simulink model "missionplanning"  (R2020b)
settings: Solver=FixedStepAuto  StartTime=0.0  StopTime=10.0  FixedStep=0.1  RelTol=1e-3
values from neighbouring files (symbols this model uses):
  A_DB = euler2A(1,1,1,45*pi/180,0,0)    [main.m]
libraries: aerolibtransform2 x1
settings Model: Creator=tjones  LastModifiedBy=tjones

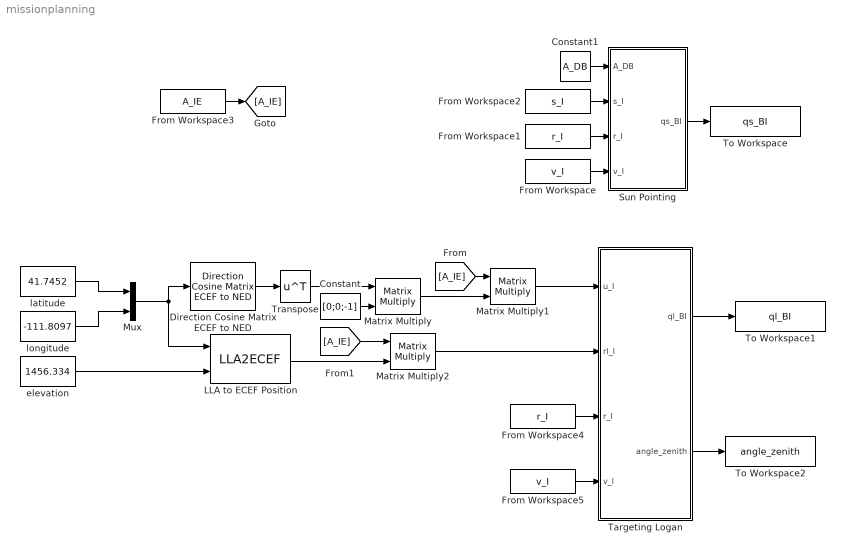
== system missionplanning ==
  Constant : Constant  Value=[0;0;-1]
  Constant1 : Constant  Value=A_DB
  Direction Cosine Matrix ECEF to NED : aerolibtransform2/Direction Cosine Matrix ECEF to NED
      settings: SourceProductBaseCode=AE
  From Workspace : FromWorkspace  VariableName=v_I
  From Workspace1 : FromWorkspace  VariableName=r_I
  From Workspace2 : FromWorkspace  VariableName=s_I
  From Workspace3 : FromWorkspace  VariableName=A_IE
  From Workspace4 : FromWorkspace  VariableName=r_I
  From Workspace5 : FromWorkspace  VariableName=v_I
  LLA to ECEF Position : LLA2ECEF
  Matrix Multiply : Product  Multiplication=Matrix(*)
  Matrix Multiply1 : Product  Multiplication=Matrix(*)
  Matrix Multiply2 : Product  Multiplication=Matrix(*)
  Mux : Mux  Inputs=2
  Sun Pointing : MATLAB Function  TreatAsAtomicUnit=on
  Targeting Logan : MATLAB Function  TreatAsAtomicUnit=on
  To Workspace : ToWorkspace  VariableName=qs_BI  SaveFormat=Timeseries  SampleTime=-1
  To Workspace1 : ToWorkspace  VariableName=ql_BI  SaveFormat=Timeseries  SampleTime=-1
  To Workspace2 : ToWorkspace  VariableName=angle_zenith  SaveFormat=Timeseries  SampleTime=-1
  Transpose : Math  Operator=transpose  SaturateOnIntegerOverflow=on
  elevation : Constant  Value=1456.334
  latitude : Constant  Value=41.7452
  longitude : Constant  Value=-111.8097
  wires:
  latitude/1 -> Mux/1
  longitude/1 -> Mux/2
  Mux/1 -> LLA to ECEF Position/1, Direction Cosine Matrix ECEF to NED/1
  Direction Cosine Matrix ECEF to NED/1 -> Transpose/1
  Transpose/1 -> Matrix Multiply/1
  Constant/1 -> Matrix Multiply/2
  Matrix Multiply/1 -> Matrix Multiply1/2
  [A_IE] -> Matrix Multiply1/1
  Matrix Multiply1/1 -> Targeting Logan/1(u_I)
  elevation/1 -> LLA to ECEF Position/2
  [A_IE] -> Matrix Multiply2/1
  LLA to ECEF Position/1 -> Matrix Multiply2/2
  Matrix Multiply2/1 -> Targeting Logan/2(rl_I)
  From Workspace/1 -> Sun Pointing/4(v_I)
  From Workspace1/1 -> Sun Pointing/3(r_I)
  From Workspace2/1 -> Sun Pointing/2(s_I)
  From Workspace3/1 -> [A_IE]
  Constant1/1 -> Sun Pointing/1(A_DB)
  Sun Pointing/1(qs_BI) -> To Workspace/1
  Targeting Logan/1(ql_BI) -> To Workspace1/1
  Targeting Logan/2(angle_zenith) -> To Workspace2/1
  From Workspace4/1 -> Targeting Logan/3(r_I)
  From Workspace5/1 -> Targeting Logan/4(v_I)

== matlab function missionplanning/Targeting Logan ==
  data: u_I input; ql_BI output Bus: qBus; rl_I input; r_I input; v_I input; angle_zenith output
function [ql_BI, angle_zenith] = fcn(u_I, rl_I, r_I, v_I)

[ql_BI, angle_zenith] = groundTarget(u_I, rl_I, r_I, v_I);

== matlab function missionplanning/Sun Pointing ==
  data: A_DB input; qs_BI output Bus: qBus; s_I input; r_I input; v_I input
function qs_BI = fcn(A_DB, s_I, r_I, v_I)

% vector from spacecraft to sun
ss_I = s_I - r_I;

% Point Y Basis of Deployed at Sun
yd_I = ss_I/norm(ss_I);

% Calculate Unit Angular Momentum Vector
h_I = cross(r_I,v_I);
h_I = h_I/norm(h_I);

% Indirectly satisfy Secondary constraint
zd_I = cross(h_I, yd_I);
zd_I = zd_I/norm(zd_I);

% Complete the triad
xd_I = cross(yd_I, zd_I);
xd_I = xd_I/norm(xd_I);

% DCM from Inertial to Deployed
A_DI = [xd_I'; yd_I'; zd_I'];

A_BD = A_DB';

% Create inertial to body DCM
A_BI = A_BD*A_DI;

% Desired Quaternion to Point at the sun
qs_BI = A2q(A_BI);
